simulink model "Test_Models"  (R2022a)
settings: Solver=VariableStepAuto  StartTime=0.0  StopTime=10.0  RelTol=1e-3
settings Model: Creator=aasav  LastModifiedBy=aasav

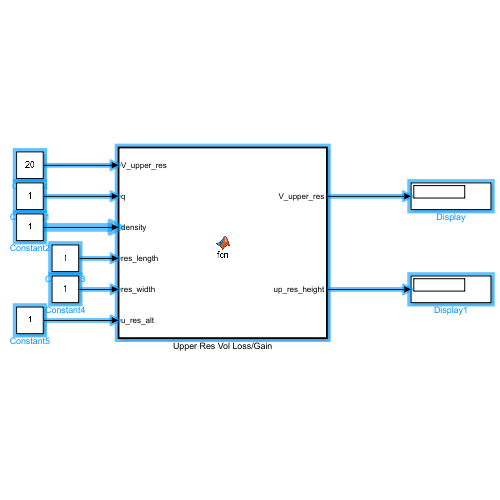
[thumbnail: Simulink's stored preview of the top-level diagram]
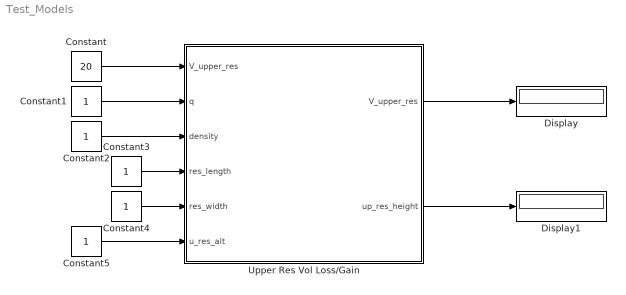
== system Test_Models ==
  Constant : Constant  Value=20
  Constant{1..5} (5 alike) : Constant
  Display : Display
  Display1 : Display
  Upper Res Vol Loss/Gain : MATLAB Function  TreatAsAtomicUnit=on
  wires:
  Constant/1 -> Upper Res Vol Loss/Gain/1("V_upper_res ")
  Constant1/1 -> Upper Res Vol Loss/Gain/2(q)
  Upper Res Vol Loss/Gain/2(up_res_height) -> Display1/1
  Constant3/1 -> Upper Res Vol Loss/Gain/4(res_length)
  Constant5/1 -> Upper Res Vol Loss/Gain/6(u_res_alt)
  Upper Res Vol Loss/Gain/1(V_upper_res) -> Display/1
  Constant4/1 -> Upper Res Vol Loss/Gain/5(res_width)
  Constant2/1 -> Upper Res Vol Loss/Gain/3(density)

== matlab function Test_Models/Upper Res Vol Loss//Gain ==
  data: V_upper_res output; V_upper_res input; q input; density input; res_length input; res_width input; up_res_height output; u_res_alt input
function [V_upper_res, up_res_height] = fcn(V_upper_res, q, density, res_length, res_width, u_res_alt)

    [V_upper_res, up_res_height] = fcn_vol_upper(V_upper_res, q, density, res_length, res_width, u_res_alt);
